simulink model "PID_c"  (R2015b)
settings: Solver=VariableStepAuto  StartTime=0.0  StopTime=10.0  RelTol=1e-3
undefined symbols (not defined in the file): D, I, N, P
settings Model: Creator=mgreiff  LastModifiedBy=mgreiff

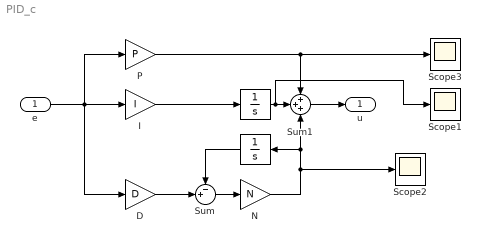
== system PID_c ==
  e : Inport
  " " : Integrator
  "   " : Integrator
  D : Gain  Gain=D
  I : Gain  Gain=I
  N : Gain  Gain=N
  P : Gain  Gain=P
  Scope1 : Scope
  Scope2 : Scope
  Scope3 : Scope
  Sum : Sum  Inputs=-+|
  Sum1 : Sum  Inputs=+++
  u : Outport
  wires:
  e/1 -> D/1, P/1, I/1
  D/1 -> Sum/2
  Sum/1 -> N/1
  I/1 -> " "/1
  N/1 -> Sum1/3, "   "/1, Scope2/1
  "   "/1 -> Sum/1
  P/1 -> Scope3/1, Sum1/1
  " "/1 -> Scope1/1, Sum1/2
  Sum1/1 -> u/1
